simulink model "FOC"  (R2023a)
settings: Solver=VariableStepAuto  StartTime=0.0  StopTime=10.0  RelTol=1e-3
libraries: ee_lib x1
settings Model: Creator=xuluyu  LastModifiedBy=xuluyu

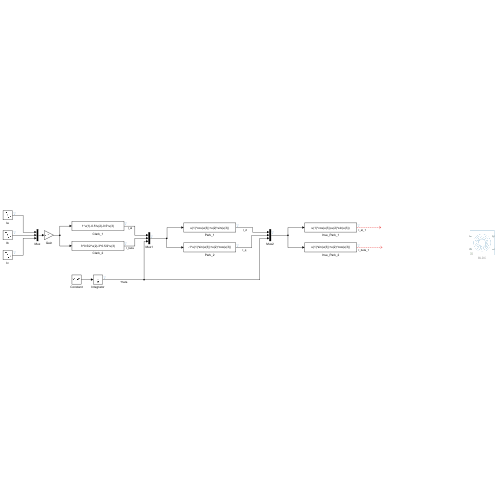
[thumbnail: Simulink's stored preview of the top-level diagram]
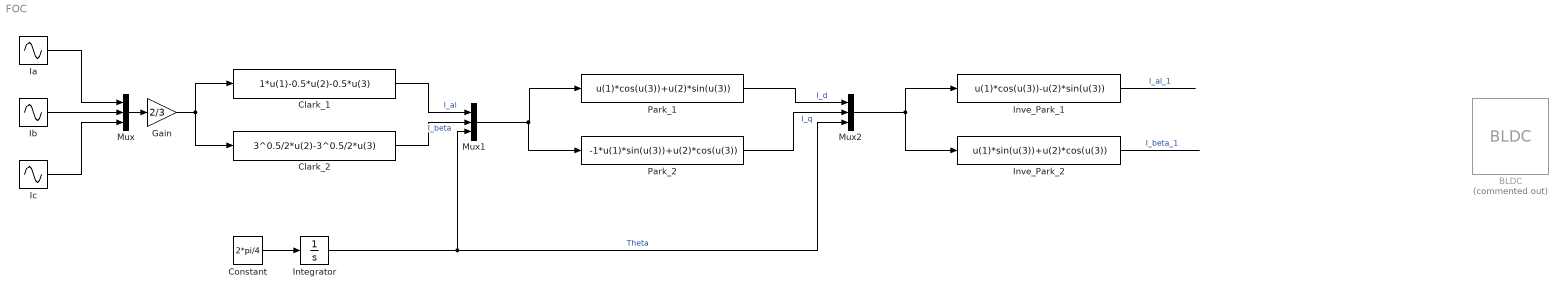
== system FOC ==
  BLDC : ee_lib/Electromechanical/Permanent Magnet/BLDC  Commented=on  port_option=ee.enum.threePhasePort.composite  winding_type=ee.enum.statorconnection.wye  rotor_param=ee.enum.pmsm.backemf.trapezoidflux  pm_flux_linkage=0.03 Wb  theta_constant=pi / 12 rad  emf_max=9.6 V  w_meas=600 rpm  DphiDtheta_tab=[0, -.1528, -.1528, .1528, .1528, 0] Wb/rad  back_emf_tab=[0, -9.6, -9.6, 9.6, 9.6, 0] V  rotor_angle_tab=[0, 7.5, 22.5, 37.5, 52.5, 60] deg  nPolePairs=6  axes_param=ee.enum.rotorangle.daxis  stator_param=ee.enum.statorparam.LdLqL0  machine_param=ee.enum.dqparameterization.constant  Ld=0.00022 H  Lq=0.00022 H  idVec=[-200, 0, 200] A  iqVec=[-200, 0, 200] A  LdMatrix=0.00022 * ones(3, 3) H  LqMatrix=0.00022 * ones(3, 3) H  L0=0.00016 H  Ls=0.0002 H  Lm=0 H  Ms=0.00002 H  Rs=0.013 Ohm  zero_sequence=ee.enum.park.zerosequence.include  loss_param=ee.enum.ironloss.none  losses_oc=[0, 0, 0] W  losses_sc=[0, 0, 0] W  f_losses=60 Hz  Isc_losses=95 A  J=0.01 kg*m^2  lam=0 N*m*s/rad  i_d_specify=off  i_d_priority=None  i_d=0 A  i_d_nominal_specify=off  i_d_nominal_unit=A  i_d_nominal_value=1  i_q_specify=off  i_q_priority=None  i_q=0 A  i_q_nominal_specify=off  i_q_nominal_unit=A  i_q_nominal_value=1  torque_specify=off  torque_priority=None  torque=0 N*m  torque_nominal_specify=off  torque_nominal_unit=N*m  torque_nominal_value=1  angular_velocity_specify=off  angular_velocity_priority=High  angular_velocity=0 rpm  angular_velocity_nominal_specify=off  angular_velocity_nominal_unit=rpm  angular_velocity_nominal_value=1  angular_position_specify=off  angular_position_priority=High  angular_position=0 deg  angular_position_nominal_specify=off  angular_position_nominal_unit=deg  angular_position_nominal_value=1  alpha=3.93e-3 1/K  alpha_flux=-0.001 1/K  Tmeas=298.15 K  stator_thermal_mass=100 J/K  rotor_thermal_mass=200 J/K  Rm_percent_rotor=90  Rd_percent_rotor=30  temperatureA_specify=off  temperatureA_priority=High  temperatureA=25 degC  temperatureA_nominal_specify=off  temperatureA_nominal_unit=degC  temperatureA_nominal_value=1  temperatureB_specify=off  temperatureB_priority=High  temperatureB=25 degC  temperatureB_nominal_specify=off  temperatureB_nominal_unit=degC  temperatureB_nominal_value=1  temperatureC_specify=off  temperatureC_priority=High  temperatureC=25 degC  temperatureC_nominal_specify=off  temperatureC_nominal_unit=degC  temperatureC_nominal_value=1  temperatureR_specify=off  temperatureR_priority=High  temperatureR=25 degC  temperatureR_nominal_specify=off  temperatureR_nominal_unit=degC  temperatureR_nominal_value=1
      settings: InternalSimscapePortConfiguration="{\"Bottom\":[],\"Left\":[{\"id\":\"N\",\"label\":\"~\",\"type\":\"foundation.electrical.three_phase\"},{\"id\":\"n\",\"label\":\"n\",\"type\":\"foundation.electrical.electrical\"}],\"Right\":[{\"id\":\"R\",\"label\":\"R\",\"type\":\"foundation.mechanical.rotational.rotational\"},{\"id\":\"C\",\"label\":\"C\",\"type\":\"foundation.mechanical.rotational.rotational\"}],\"Top\":[]}"
  Clark_1 : Fcn  Expr=1*u(1)-0.5*u(2)-0.5*u(3)
  Clark_2 : Fcn  Expr=3^0.5/2*u(2)-3^0.5/2*u(3)
  Constant : Constant  Value=2*pi/4
  Gain : Gain  Gain=2/3
  Ia : Sin  Frequency=2*pi/4  Phase=0+pi/2  SampleTime=0
  Ib : Sin  Frequency=2*pi/4  Phase=-2*pi/3+pi/2  SampleTime=0
  Ic : Sin  Frequency=2*pi/4  Phase=+2*pi/3+pi/2  SampleTime=0
  Integrator : Integrator
  Inve_Park_1 : Fcn  Expr=u(1)*cos(u(3))-u(2)*sin(u(3))
  Inve_Park_2 : Fcn  Expr=u(1)*sin(u(3))+u(2)*cos(u(3))
  Mux : Mux  Inputs=3
  Mux1 : Mux  Inputs=3
  Mux2 : Mux  Inputs=3
  Park_1 : Fcn  Expr=u(1)*cos(u(3))+u(2)*sin(u(3))
  Park_2 : Fcn  Expr=-1*u(1)*sin(u(3))+u(2)*cos(u(3))
  wires:
  Mux/1 -> Gain/1
  Ia/1 -> Mux/1
  Ib/1 -> Mux/2
  Ic/1 -> Mux/3
  Clark_1/1 -> Mux1/1  "I_al"
  Clark_2/1 -> Mux1/2  "I_beta"
  Gain/1 -> Clark_2/1, Clark_1/1
  Constant/1 -> Integrator/1
  Integrator/1 -> Mux2/3, Mux1/3  "Theta"
  Mux1/1 -> Park_2/1, Park_1/1
  Park_1/1 -> Mux2/1  "I_d"
  Park_2/1 -> Mux2/2  "I_q"
  Mux2/1 -> Inve_Park_2/1, Inve_Park_1/1
  Inve_Park_1/1 -> ?  "I_al_1"
  Inve_Park_2/1 -> ?  "I_beta_1"
